simulink model "Subsystem"  (R2020b)
settings: Solver=FixedStepAuto  StartTime=0.0  StopTime=3  FixedStep=0.06  RelTol=1e-3
settings Model: Creator=shubham sharma  LastModifiedBy=shubham sharma
settings DataIOCC: SaveOutput=off  SaveTime=off

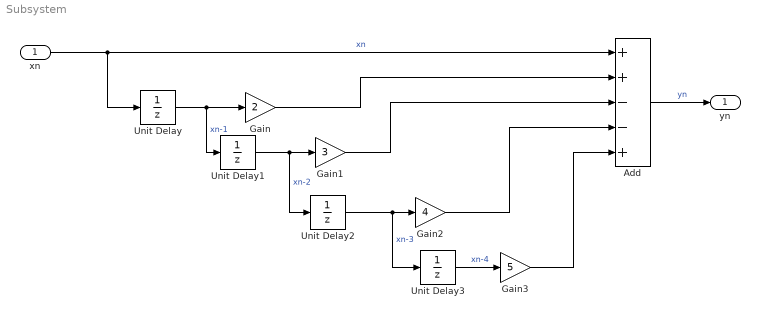
== system Subsystem ==
  xn : Inport  OutDataTypeStr=double  PortDimensions=1
  Add : Sum  Inputs=++--+
  Gain : Gain  Gain=2
  Gain1 : Gain  Gain=3
  Gain2 : Gain  Gain=4
  Gain3 : Gain  Gain=5
  Unit Delay{,1..3} (4 alike) : UnitDelay  SampleTime=-1  HasFrameUpgradeWarning=on
  yn : Outport  OutDataTypeStr=double  PortDimensions=1  SampleTime=[0.059999999999999998,0]
  wires:
  xn/1 -> Add/1, Unit Delay/1  "xn"
  Unit Delay1/1 -> Gain1/1, Unit Delay2/1  "xn-2"
  Gain2/1 -> Add/4
  Unit Delay/1 -> Gain/1, Unit Delay1/1  "xn-1"
  Gain1/1 -> Add/3
  Unit Delay2/1 -> Gain2/1, Unit Delay3/1  "xn-3"
  Gain/1 -> Add/2
  Unit Delay3/1 -> Gain3/1  "xn-4"
  Gain3/1 -> Add/5
  Add/1 -> yn/1  "yn"
